simulink model "ifelse"  (R2019a)
settings: Solver=VariableStepAuto  StartTime=0.0  StopTime=10.0  RelTol=1e-3
settings Model: Creator=victor  LastModifiedBy=victor

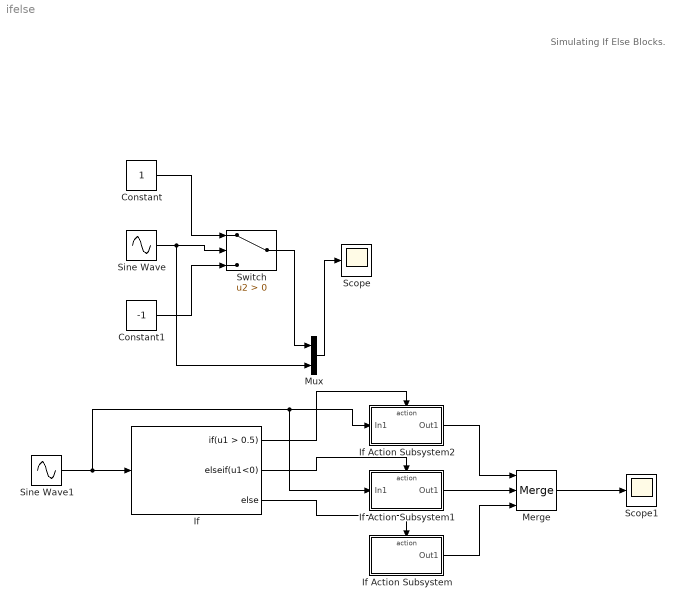
== system ifelse ==
  note: Simulating If Else Blocks.
  Constant : Constant
  Constant1 : Constant  Value=-1
  If : If  IfExpression=u1 > 0.5  ElseIfExpressions=u1<0
  If Action Subsystem : Subsystem  TreatAsAtomicUnit=on
  If Action Subsystem1 : Subsystem  TreatAsAtomicUnit=on
  If Action Subsystem2 : Subsystem  TreatAsAtomicUnit=on
  Merge : Merge  Inputs=3
  Mux : Mux  Inputs=2
  Scope : Scope
  Scope1 : Scope
  Sine Wave : Sin  SampleTime=0
  Sine Wave1 : Sin  SampleTime=0
  Switch : Switch  Criteria=u2 > Threshold
  wires:
  Constant/1 -> Switch/1
  Constant1/1 -> Switch/3
  Sine Wave/1 -> Mux/2, Switch/2
  Switch/1 -> Mux/1
  Mux/1 -> Scope/1
  Sine Wave1/1 -> If Action Subsystem1/1(In1), If Action Subsystem2/1(In1), If/1
  If/1 -> If Action Subsystem2/Action
  If/2 -> If Action Subsystem1/Action
  If/3 -> If Action Subsystem/Action
  If Action Subsystem2/1(Out1) -> Merge/1
  If Action Subsystem1/1(Out1) -> Merge/2
  If Action Subsystem/1(Out1) -> Merge/3
  Merge/1 -> Scope1/1

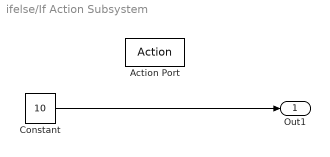
== system ifelse/If Action Subsystem ==
  Action Port : ActionPort  ActionPortLabel=else
  Constant : Constant  Value=10
  Out1 : Outport
  wires:
  Constant/1 -> Out1/1

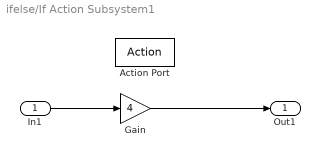
== system ifelse/If Action Subsystem1 ==
  In1 : Inport
  Action Port : ActionPort  ActionPortLabel=elseif(u1<0)
  Gain : Gain  Gain=4
  Out1 : Outport
  wires:
  In1/1 -> Gain/1
  Gain/1 -> Out1/1

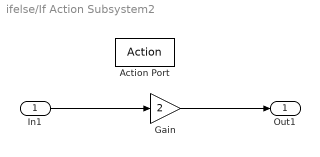
== system ifelse/If Action Subsystem2 ==
  In1 : Inport
  Action Port : ActionPort  ActionPortLabel=if(u1 > 0.5)
  Gain : Gain  Gain=2
  Out1 : Outport
  wires:
  In1/1 -> Gain/1
  Gain/1 -> Out1/1
